simulink model "Rail"  (R2018a)
settings: configuration reference "cs_ert" (kept outside this file)
settings Model: DataDictionary=Rail.sldd  Creator=zhoutinglin  LastModifiedBy=zhoutinglin

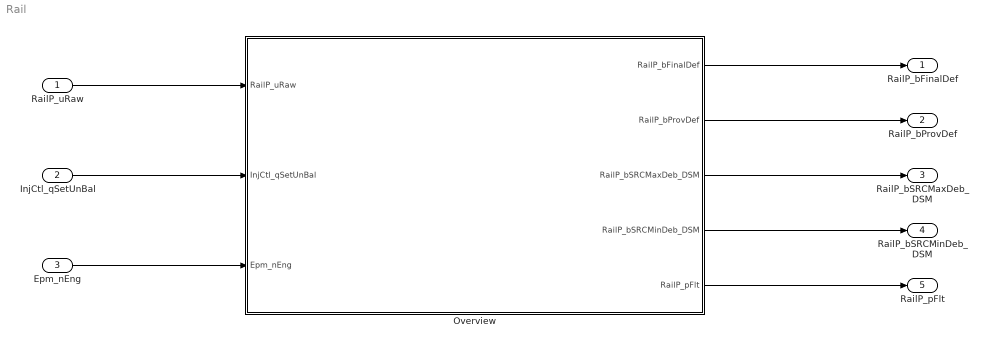
== system Rail ==
  RailP_uRaw : Inport
  InjCtl_qSetUnBal : Inport  Port=2
  Epm_nEng : Inport  Port=3
  Overview : Subsystem
  RailP_bFinalDef : Outport
  RailP_bProvDef : Outport  Port=2
  RailP_bSRCMaxDeb_DSM : Outport  Port=3
  RailP_bSRCMinDeb_DSM : Outport  Port=4
  RailP_pFlt : Outport  Port=5
  wires:
  RailP_uRaw/1 -> Overview/1(RailP_uRaw)
  InjCtl_qSetUnBal/1 -> Overview/2(InjCtl_qSetUnBal)
  Epm_nEng/1 -> Overview/3(Epm_nEng)
  Overview/1(RailP_bFinalDef) -> RailP_bFinalDef/1
  Overview/2(RailP_bProvDef) -> RailP_bProvDef/1
  Overview/3(RailP_bSRCMaxDeb_DSM) -> RailP_bSRCMaxDeb_DSM/1
  Overview/4(RailP_bSRCMinDeb_DSM) -> RailP_bSRCMinDeb_DSM/1
  Overview/5(RailP_pFlt) -> RailP_pFlt/1

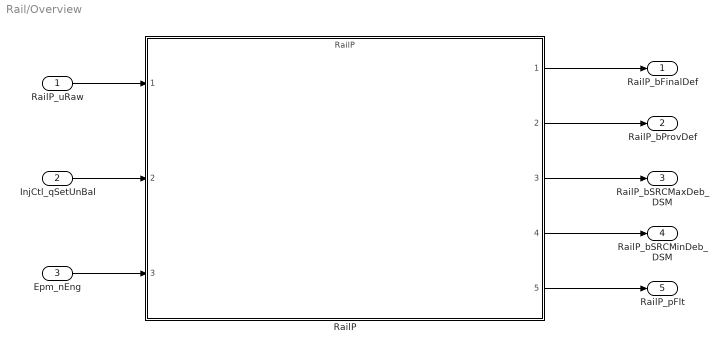
== system Rail/Overview ==
  RailP_uRaw : Inport
  InjCtl_qSetUnBal : Inport  Port=2
  Epm_nEng : Inport  Port=3
  RailP : ModelReference  ModelNameDialog=RailP  SimulationMode=Normal  ModelReferenceVersion=1.4
  RailP_bFinalDef : Outport
  RailP_bProvDef : Outport  Port=2
  RailP_bSRCMaxDeb_DSM : Outport  Port=3
  RailP_bSRCMinDeb_DSM : Outport  Port=4
  RailP_pFlt : Outport  Port=5
  wires:
  RailP_uRaw/1 -> RailP/1
  InjCtl_qSetUnBal/1 -> RailP/2
  Epm_nEng/1 -> RailP/3
  RailP/1 -> RailP_bFinalDef/1
  RailP/2 -> RailP_bProvDef/1
  RailP/3 -> RailP_bSRCMaxDeb_DSM/1
  RailP/4 -> RailP_bSRCMinDeb_DSM/1
  RailP/5 -> RailP_pFlt/1
